simulink model "systemModel_Final"  (R2022a)
settings: Solver=ode3  StartTime=0.0  StopTime=3  FixedStep=0.01  RelTol=1e-3  EnableMultiTasking=on
libraries: fuzblock x1
settings Model: Creator=Φίλιππος  LastModifiedBy=user1
settings SolverCC: AlgebraicLoopSolver=TrustRegion
settings DataIOCC: LimitDataPoints=on  SaveFormat=Array  ReturnWorkspaceOutputs=off
settings OptimizationCC: LifeSpan=inf
settings DebuggingCC: UnconnectedInputMsg=warning  UnconnectedOutputMsg=warning  UnconnectedLineMsg=warning  SFUnexpectedBacktrackingDiag=warning  SFNoUnconditionalDefaultTransitionDiag=warning  SFExecutionAtInitializationDiag=none  SFMachineParentedDataDiag=warning  ArithmeticOperatorsInVariantConditions=warning
settings HardwareCC: ProdBitPerPointer=32  ProdBitPerSizeT=32  ProdBitPerPtrDiffT=32  ProdLargestAtomicFloat=None  ProdIntDivRoundTo=Undefined  ProdEndianess=Unspecified  ProdWordSize=32  ProdHWDeviceType=32-bit Generic
settings ModelReferenceCC: PropagateSignalLabelsOutOfModel=off
settings SFSimCC: SimUseLocalCustomCode=off  CustomCodeUndefinedFunction=UseInterfaceOnly
settings RTWCC: RTWUseLocalCustomCode=off
settings CodeAppCC: StateflowObjectComments=on
settings GRTTargetCC: TargetLangStandard=C89/C90 (ANSI)
settings ConfigComp: CovMetricSettings=dw  CovSaveCumulativeToWorkspaceVar=on  CovSaveSingleToWorkspaceVar=on  CovExternalEMLEnable=off  DVMaxTestCaseSteps=500  DVTestSuiteOptimization=CombinedObjectives (Nonlinear Extended)  DVHarnessSource=Signal Editor

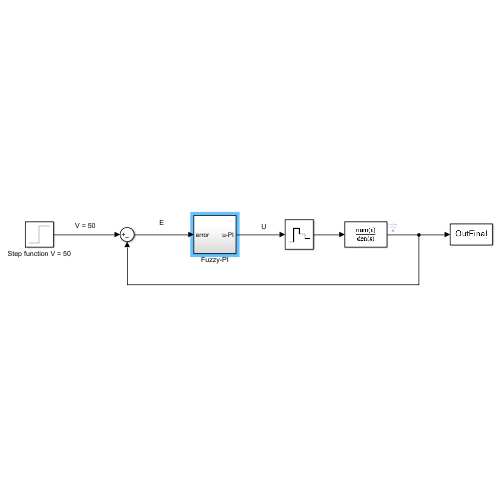
[thumbnail: Simulink's stored preview of the top-level diagram]
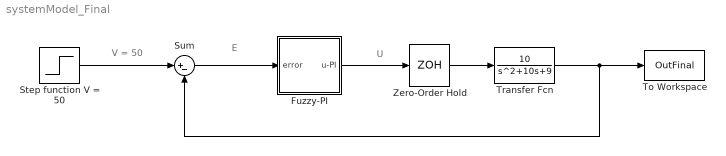
== system systemModel_Final ==
  note: U
  note: E
  note: V = 50
  Fuzzy-PI : Subsystem
  Step function V = 50 : Step  Time=0  After=50  SampleTime=0  ZeroCross=off
  Sum : Sum  Inputs=|+-
  To Workspace : ToWorkspace  VariableName=OutFinal  SaveFormat=Timeseries  SampleTime=-1
  Transfer Fcn : TransferFcn  Numerator=[10]  Denominator=[1 10 9]
  Zero-Order Hold : ZeroOrderHold  SampleTime=0.01
  wires:
  Zero-Order Hold/1 -> Transfer Fcn/1
  Step function V = 50/1 -> Sum/1
  Transfer Fcn/1 -> To Workspace/1, Sum/2
  Fuzzy-PI/1(u-PI) -> Zero-Order Hold/1
  Sum/1 -> Fuzzy-PI/1(error)

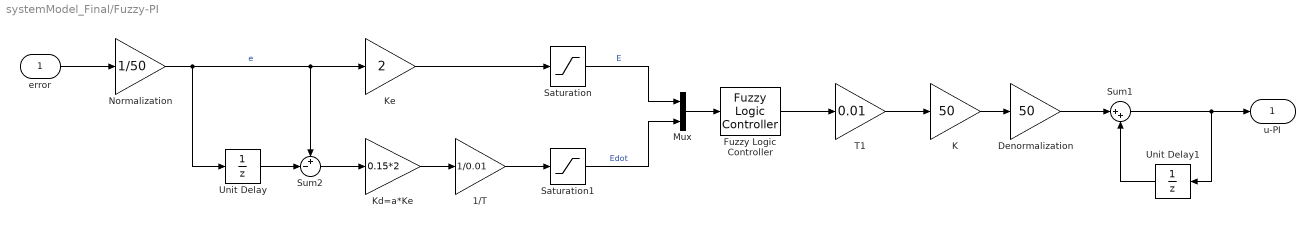
== system systemModel_Final/Fuzzy-PI ==
  error : Inport
  1/T : Gain  Gain=1/0.01
  Denormalization : Gain  Gain=50
  Fuzzy Logic Controller : fuzblock/Fuzzy Logic  Controller  FIS='FuzzyController.fis'  OutputSampleNumber=101  DataType=double  FuzzifiedInputs=off  RuleFiringStrengths=off  RuleOutputs=off  AggregatedOutputs=off  SimulateUsing=Interpreted execution  OutOfRangeInputValueMessage=warning  NoRuleFiredMessage=warning  EmptyOutputFuzzySetMessage=warning
  K : Gain  Gain=50
  Kd=a*Ke : Gain  Gain=0.15*2
  Ke : Gain  Gain=2
  Mux : Mux  Inputs=2
  Normalization : Gain  Gain=1/50
  Saturation : Saturate  UpperLimit=1  LowerLimit=-1
  Saturation1 : Saturate  UpperLimit=1  LowerLimit=-1
  Sum1 : Sum  Inputs=|++
  Sum2 : Sum  Inputs=+-|
  T1 : Gain  Gain=0.01
  Unit Delay : UnitDelay  SampleTime=-1  HasFrameUpgradeWarning=on
  Unit Delay1 : UnitDelay  SampleTime=-1  HasFrameUpgradeWarning=on
  u-PI : Outport
  wires:
  error/1 -> Normalization/1
  Normalization/1 -> Unit Delay/1, Sum2/1, Ke/1  "e"
  Unit Delay/1 -> Sum2/2
  Ke/1 -> Saturation/1
  Kd=a*Ke/1 -> 1/T/1
  1/T/1 -> Saturation1/1
  Saturation/1 -> Mux/1  "E"
  Saturation1/1 -> Mux/2  "Edot"
  Mux/1 -> Fuzzy Logic Controller/1
  Fuzzy Logic Controller/1 -> T1/1
  T1/1 -> K/1
  K/1 -> Denormalization/1
  Denormalization/1 -> Sum1/1
  Sum1/1 -> Unit Delay1/1, u-PI/1
  Unit Delay1/1 -> Sum1/2
  Sum2/1 -> Kd=a*Ke/1
